simulink model "gyroNoiseStudy"  (R2017b)
settings: Solver=VariableStepAuto  StartTime=0.0  StopTime=time(end)  RelTol=1e-3
undefined symbols (not defined in the file): ST
settings Model: Creator=CC  LastModifiedBy=CC

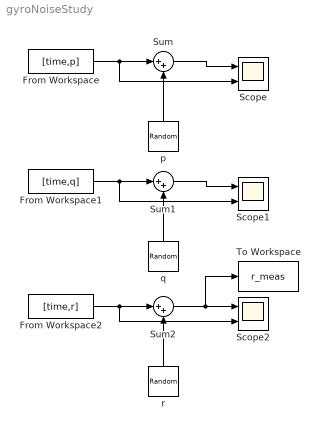
== system gyroNoiseStudy ==
  From Workspace : FromWorkspace  VariableName=[time,p]  OutDataTypeStr=double  SampleTime=0
  From Workspace1 : FromWorkspace  VariableName=[time,q]  OutDataTypeStr=double  SampleTime=0
  From Workspace2 : FromWorkspace  VariableName=[time,r]  OutDataTypeStr=double  SampleTime=0
  Scope : Scope  NumInputPorts=2
  Scope1 : Scope  NumInputPorts=2
  Scope2 : Scope  NumInputPorts=2
  Sum : Sum  Inputs=|++
  Sum1 : Sum  Inputs=|++
  Sum2 : Sum  Inputs=|++
  To Workspace : ToWorkspace  VariableName=r_meas  SampleTime=-1
  p : RandomNumber  Variance=0.005  SampleTime=ST
  q : RandomNumber  Variance=0.005  SampleTime=ST
  r : RandomNumber  Variance=0.005  SampleTime=ST
  wires:
  From Workspace/1 -> Scope/2, Sum/1
  Sum/1 -> Scope/1
  p/1 -> Sum/2
  From Workspace1/1 -> Scope1/2, Sum1/1
  q/1 -> Sum1/2
  Sum1/1 -> Scope1/1
  r/1 -> Sum2/2
  Sum2/1 -> To Workspace/1, Scope2/1
  From Workspace2/1 -> Scope2/2, Sum2/1
